simulink library "Collector_Unglazed_ISO_2node"  (R2018b)
settings: Solver=ode45  StartTime=0.0  StopTime=10.0  RelTol=1e-3  EnableMultiTasking=on
undefined symbols (not defined in the file): path_carnot
libraries: carnot x5
settings Model: Creator=drhf  LastModifiedBy=drhf
settings DataIOCC: LimitDataPoints=on  SaveFormat=Array  SignalLoggingSaveFormat=ModelDataLogs
settings OptimizationCC: ExpressionDepthLimit=2147483647  LifeSpan=inf
settings DebuggingCC: UnderspecifiedInitializationDetection=Classic  MergeDetectMultiDrivingBlocksExec=none  SolverPrmCheckMsg=warning  FcnCallInpInsideContextMsg=warning  StateNameClashWarn=warning  SFUnexpectedBacktrackingDiag=warning  SFNoUnconditionalDefaultTransitionDiag=warning  SFExecutionAtInitializationDiag=none
settings HardwareCC: ProdBitPerPointer=32  ProdBitPerSizeT=32  ProdBitPerPtrDiffT=32  ProdLargestAtomicFloat=None  ProdIntDivRoundTo=Undefined  ProdEndianess=Unspecified  ProdWordSize=32  ProdHWDeviceType=32-bit Generic
settings ModelReferenceCC: PropagateSignalLabelsOutOfModel=off
settings SFSimCC: SimUseLocalCustomCode=off
settings RTWCC: RTWUseLocalCustomCode=off
settings CodeAppCC: StateflowObjectComments=on
settings GRTTargetCC: TargetLangStandard=C89/C90 (ANSI)  GeneratePreprocessorConditionals=Disable all  CombineOutputUpdateFcns=off  GRTInterface=on
settings ConfigComp: CovMetricSettings=dw  CovHtmlReporting=on  CovSaveCumulativeToWorkspaceVar=on  CovSaveSingleToWorkspaceVar=on  CovExternalEMLEnable=off

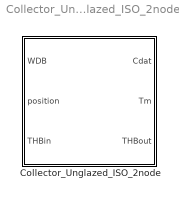
== system Collector_Unglazed_ISO_2node ==
  Collector_Unglazed_ISO_2node : Subsystem  mask(Unglazed solar thermal collector){tini=20, Ncollector=1, PathName=fullfile(path_carnot('libsl'), 'Source', 'Solar_Thermal', 'Collector_Unglazed_ISO9806', 'parameter_set'), FileName='Viessmann_SLK_ISO9806.mat', userPath=off, userParam=off, acol=2.544, len=2.1, eta0=0.702, bu=0.066, b1=32.64, b2=3.59, c_abs=50*3900, dplin=5504.4, dpqua=6222.096}
      mask prompts: tini "Initial temperature [°C]"; Ncollector "Number of collectors in parallel"; PathName "Path"; FileName "Parameter set"; userPath "Edit path and name of parameter set"; userParam "User defined parameters"; acol "Collector surface (aperture) in [m²]"; len "Length between inlet and outlet [m]"; eta0 "Optical efficiency Eta0 [-]"; bu "bu: wind dependancy of optical efficiency in W/(m²*m/s)"; b1 "b1: heat transfer for losses [W/(m²*K)]"; b2 "b2: wind dependent heat transfer for losses [W/(m²*K*m/s)]"; c_abs "Effective heat capacity of absorber [J/(m²*K)]"; dplin "Linear pressure drop in Pa/(kg/s)"; dpqua "Quadratic pressure drop in Pa/(kg/s)²"
      mask help:
      | Modified ISO 9806 model of an unglazed solar thermal collector with 2 thermal capacity nodes. The first thermal node is at the inlet, the second node is at the oulet. Both nodes have half of the capacity of the ISO test report.
      |  Qdot = A*G*(eta0*(1-bu*vwind) - (b1 + b2*vwind)*(Tm-Tamb)/G)
      |  Qdot = mdot*cp*(Tout-Tin)
      |  Tm = (Tout+Tin)/2
      |  dTin/dt = mdot*cp*(Tinlet-Tin)*2/(Acol*Ncol*CapAbs)
      |  dTout/dt = (-mdot*cp*(Tout-Tin)/(Acol*Ncol) + (G*eta0*(1-bu*vwind) - (b1 + b2*vwind)*(Tm-Tamb)))*2/CapAbs
      | This modified equations respect energy conservation also for variable inlet conditions (e.g. temperature).
      | IT IS RECOMMENDED TO USE THIS MODEL FOR SYSTEM SIMULATIONS (instead of the Collector Unglazed ISO 9806 model).
      mask init:
      | % callback to set parameters of model
      | [ok, param] = CarnotCallbacks_CONFblocksMain('SetParameters',gcbh,PathName,FileName, ...
      |     fullfile('Source','Solar_Thermal','Collector_Unglazed_ISO_2node','parameter_set'));
      | 
      | % [ok, param] = CarnotCallbacks_CollectorUnglazedConf('SetParameters',gcbh,PathName,FileName);
      mask Help: web(fullfile(path_carnot('help'),'Collector_Unglazed_ISO_2node.html'),'-helpbrowser')
      mask TypeOptions tini: Integrator/InitialCondition | Tin_node/Integrator/InitialCondition
      mask TypeOptions Ncollector: ncol/Gain | Pressure Drop/Ncoll/Value
      mask Callback userPath:
      | [ok, param] = CarnotCallbacks_CONFblocksMain('UserEdit',gcbh,...
      |     'userPath','userParam','FileName');
      mask Callback userParam: [ok, param] = CarnotCallbacks_CONFblocksMain('UserEdit',gcbh,'userPath','userParam','FileName');
      mask TypeOptions acol: acol/Value
      mask TypeOptions len: Pressure Drop/Pressure_Drop_Collector/len
      mask TypeOptions eta0: eta0/Gain
      mask TypeOptions bu: bu/Gain
      mask TypeOptions b1: b1/Bias
      mask TypeOptions b2: b2/Gain
      mask TypeOptions c_abs: c_abs/Value
      mask TypeOptions dplin: Pressure Drop/Pressure_Drop_Collector/lin
      mask TypeOptions dpqua: Pressure Drop/Pressure_Drop_Collector/qua
      mask DialogControl Container7 Prompt: Calculation
      mask DialogControl ParameterGroupVar Prompt: Picking a parameter set
      mask DialogControl Control3 Prompt: Carnot public data
      mask DialogControl Control3 Callback:
      | [ok,file] = CarnotCallbacks_CONFblocksMain('GetFilename',gcbh, 'public', ...
      |     fullfile('Source','Solar_Thermal','Collector_Unglazed_ISO_2node','parameter_set'), ...
      |     'userPath','userParam','PathName','FileName');
      mask DialogControl Control4 Prompt: Carnot internal data
      mask DialogControl Control4 Callback:
      | [ok,file] = CarnotCallbacks_CONFblocksMain('GetFilename',gcbh, 'internal', ...
      |     fullfile('Source','Solar_Thermal','Collector_Unglazed_ISO_2node','parameter_set'), ...
      |     'userPath','userParam','PathName','FileName');
      mask DialogControl Control2 Prompt: Selected path
      mask DialogControl Control2 Callback:
      | [ok,file] = CarnotCallbacks_CONFblocksMain('GetFilename',gcbh, 'selected', ...
      |     fullfile('Source','Solar_Thermal','Collector_Unglazed_ISO_2node','parameter_set'), ...
      |     'userPath','userParam','PathName','FileName');
      mask DialogControl Container9 Prompt: Parameter values
      mask DialogControl Container8 Prompt: Geometry
      mask DialogControl Container11 Prompt: Thermal
      mask DialogControl Container12 Prompt: Hydraulic
      mask DialogControl Control6 Prompt: Save in Carnot internal data
      mask DialogControl Control6 Callback:
      | [ok, param] = CarnotCallbacks_CONFblocksMain('SaveFilename',gcbh,'internal','USTC', ...
      |     fullfile('Source','Solar_Thermal','Collector_Unglazed_ISO_2node','parameter_set'), ...
      |     'userPath','userParam','PathName','FileName');
      mask DialogControl Control5 Prompt: Save in selected path
      mask DialogControl Control5 Callback:
      | [ok, param] = CarnotCallbacks_CONFblocksMain('SaveFilename',gcbh,'selected','USTC', ...
      |     fullfile('Source','Solar_Thermal','Collector_Unglazed_ISO_2node','parameter_set'), ...
      |     'userPath','userParam','PathName','FileName');
      mask Display:
      | % user defined picture file
      | picfile = fullfile(path_carnot('intlibsl'), ...
      |     'Source','Solar_Thermal','Collector_Unglazed_ISO_2node','parameter_set','Collector_CONF.jpg');
      | 
      | pic = false;
      | 
      | % show internal picture if defined
      | if ~BlockIsInCarnotLibrary    % if not located in library any more
      |     if exist(picfile)
      |         image(imread(picfile), [0.2, 0, 0.6, 1])
      |         set_param(gcb, 'BackgroundColor', 'White')
      |         pic = true;
      |     end
      | end
      | 
      | if ~pic % show public picture
      |     disp('ISO unglazed 2 node\n\n\n\n\n\n\n\n\n\n')
      |     plot([0,70,70,0,0]/140+0.1,         [-0,-0,5,5,-0]/140+0.1, ...
      |         [30,30,100,100,30]/140+0.1,     [100,94,94,100,100]/140+0.1, ...
      |         [32,1]/140+0.1,                 [94,5]/140+0.1, ...
      |         [40,10]/140+0.1,                [94,5]/140+0.1, ...
      |         [49,19]/140+0.1,                [94,5]/140+0.1, ...
      |         [57,27]/140+0.1,                [94,5]/140+0.1, ...
      |         [65,35]/140+0.1,                [94,5]/140+0.1, ...
      |         [73,43]/140+0.1,                [94,5]/140+0.1, ...
      |         [82,51]/140+0.1,                [94,5]/140+0.1, ...
      |         [90,60]/140+0.1,                [94,5]/140+0.1,...
      |         [98,68]/140+0.1,                [94,5]/140+0.1)
      |     set_param(gcb, 'BackgroundColor', 'Yellow')
      | end

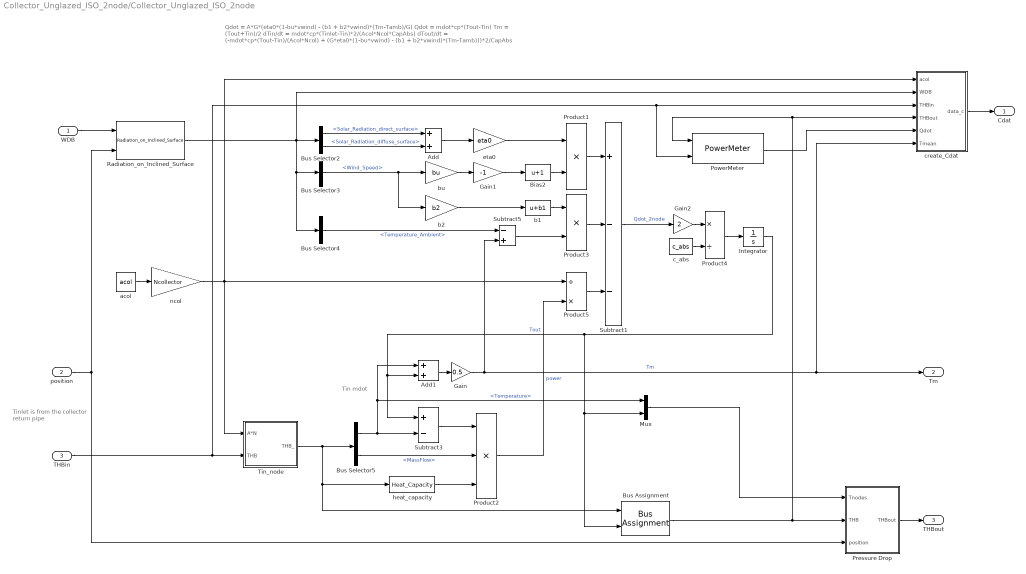
== system Collector_Unglazed_ISO_2node/Collector_Unglazed_ISO_2node ==
  note: Qdot = A*G*(eta0*(1-bu*vwind) - (b1 + b2*vwind)*(Tm-Tamb)/G)
      | Qdot = mdot*cp*(Tout-Tin)
      | Tm = (Tout+Tin)/2
      | dTin/dt = mdot*cp*(Tinlet-Tin)*2/(Acol*Ncol*CapAbs)
      | dTout/dt = (-mdot*cp*(Tout-Tin)/(Acol*Ncol) + (G*eta0*(1-bu*vwind) - (b1 + b2*vwind)*(Tm-Tamb)))*2/CapAbs
  note: Tin
      | mdot
  note: Tinlet is from the
      | collector return pipe
  WDB : Inport
  position : Inport  Port=2
  THBin : Inport  Port=3
  Add : Sum  Inputs=2
  Add1 : Sum
  Bias2 : Bias  Bias=1
  Bus Assignment : BusAssignment  AssignedSignals=Temperature
  Bus Selector2 : BusSelector  OutputSignals=Solar_Radiation_direct_surface,Solar_Radiation_diffuse_surface
  Bus Selector3 : BusSelector  OutputSignals=Wind_Speed
  Bus Selector4 : BusSelector  OutputSignals=Temperature_Ambient
  Bus Selector5 : BusSelector  OutputSignals=Temperature,MassFlow
  Gain : Gain  Gain=0.5
  Gain1 : Gain  Gain=-1
  Gain2 : Gain  Gain=2
  Integrator : Integrator  InitialCondition=tini
  Mux : Mux  Inputs=2
  PowerMeter : carnot/Control/PowerMeter
      settings: SourceProductName=Carnot
  Pressure Drop : Subsystem
  Product1 : Product  RndMeth=Zero
  Product2 : Product  Inputs=3  RndMeth=Zero
  Product3 : Product  RndMeth=Zero
  Product4 : Product  Inputs=*/  RndMeth=Zero
  Product5 : Product  Inputs=/*  RndMeth=Zero
  Radiation_on_Inclined_Surface : carnot/Weather/Radiation_on_Inclined_Surface  sky=Perez 1990  reflect=0.2
      settings: SourceProductName=Carnot
  Subtract1 : Sum  Inputs=+--
  Subtract3 : Sum  Inputs=+-
  Subtract5 : Sum  Inputs=-+
  Tin_node : Subsystem
  acol : Constant  Value=acol
  b1 : Bias  Bias=b1
  b2 : Gain  Gain=b2
  bu : Gain  Gain=bu
  c_abs : Constant  Value=c_abs
  create_Cdat : Subsystem
  eta0 : Gain  Gain=eta0
  heat_capacity : carnot/Basic/Material_Properties/Heat_Capacity  VariantControl=CarlibClassic  INPUTARGUMENTS=THB  DEBUGLEVEL=DEBUGLEVEL  MAXTOTALWARNINGS=inf  MAXCONSECUTIVEWARNINGS=inf  WRITETOFILE=0  FILENAME='errors.txt'
      settings: SourceProductName=Carnot
  ncol : Gain  Gain=Ncollector
  Cdat : Outport
  Tm : Outport  Port=2
  THBout : Outport  Port=3  InitialOutput=0
  wires:
  Gain2/1 -> Product4/1
  Mux/1 -> Pressure Drop/1(Tnodes)
  Gain/1 -> Tm/1, create_Cdat/6(Tmean), Subtract5/2  "Tm"
  Add1/1 -> Gain/1
  Integrator/1 -> Mux/2, Bus Assignment/2, Add1/2, Subtract3/1  "Tout"
  THBin/1 -> Tin_node/2(THB), PowerMeter/2, create_Cdat/3(THBin)
  Tin_node/1(THB_) -> Bus Assignment/1, heat_capacity/1, Bus Selector5/1
  Pressure Drop/1(THBout) -> THBout/1
  Product1/1 -> Subtract1/1
  Bus Selector4/1 -> Subtract5/1  "<Temperature_Ambient>"
  Bus Selector2/1 -> Add/1  "<Solar_Radiation_direct_surface>"
  Bus Selector5/1 -> Add1/1, Mux/1, Subtract3/2  "<Temperature>"
  Bus Selector2/2 -> Add/2  "<Solar_Radiation_diffuse_surface>"
  heat_capacity/1 -> Product2/3
  b2/1 -> b1/1
  Product3/1 -> Subtract1/2
  eta0/1 -> Product1/1
  Subtract5/1 -> Product3/2
  Bus Selector3/1 -> bu/1, b2/1  "<Wind_Speed>"
  b1/1 -> Product3/1
  Add/1 -> eta0/1
  Bias2/1 -> Product1/2
  Radiation_on_Inclined_Surface/1 -> Bus Selector2/1, Bus Selector3/1, Bus Selector4/1, create_Cdat/2(WDB)
  Product5/1 -> Subtract1/3
  Bus Selector5/2 -> Product2/2  "<MassFlow>"
  Subtract3/1 -> Product2/1
  Product2/1 -> Product5/2  "power"
  WDB/1 -> Radiation_on_Inclined_Surface/1
  create_Cdat/1(data_c) -> Cdat/1
  Product4/1 -> Integrator/1
  Subtract1/1 -> Gain2/1  "Qdot_2node"
  position/1 -> Pressure Drop/3(position), Radiation_on_Inclined_Surface/2
  c_abs/1 -> Product4/2
  acol/1 -> ncol/1
  bu/1 -> Gain1/1
  Bus Assignment/1 -> Pressure Drop/2(THB), create_Cdat/4(THBout), PowerMeter/1
  ncol/1 -> Tin_node/1(A*N), create_Cdat/1(acol), Product5/1
  Gain1/1 -> Bias2/1
  PowerMeter/1 -> create_Cdat/5(Qdot)

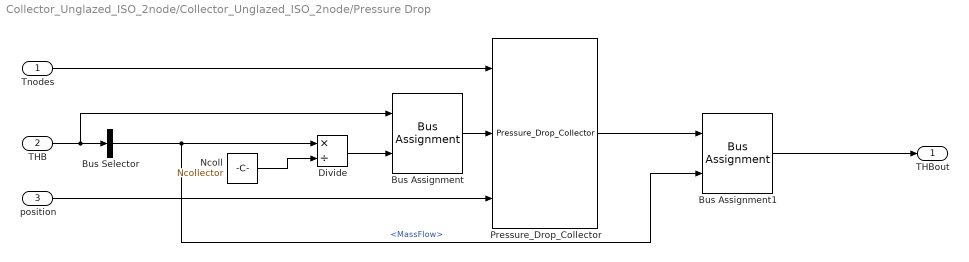
== system Collector_Unglazed_ISO_2node/Collector_Unglazed_ISO_2node/Pressure Drop ==
  Tnodes : Inport
  THB : Inport  Port=2
  position : Inport  Port=3
  Bus Assignment : BusAssignment  AssignedSignals=MassFlow
  Bus Assignment1 : BusAssignment  AssignedSignals=MassFlow
  Bus Selector : BusSelector  OutputSignals=MassFlow
  Divide : Product  Inputs=*/
  Ncoll : Constant  Value=Ncollector
  Pressure_Drop_Collector : carnot/Basic/Pressure_Drop/Pressure_Drop_Collector  len=len  lin=dplin  qua=dpqua
      settings: SourceProductName=Carnot
  THBout : Outport
  wires:
  Bus Assignment1/1 -> THBout/1
  Ncoll/1 -> Divide/2
  Divide/1 -> Bus Assignment/2
  Bus Selector/1 -> Bus Assignment1/2, Divide/1  "<MassFlow>"
  Bus Assignment/1 -> Pressure_Drop_Collector/2
  Pressure_Drop_Collector/1 -> Bus Assignment1/1
  Tnodes/1 -> Pressure_Drop_Collector/1
  position/1 -> Pressure_Drop_Collector/3
  THB/1 -> Bus Selector/1, Bus Assignment/1

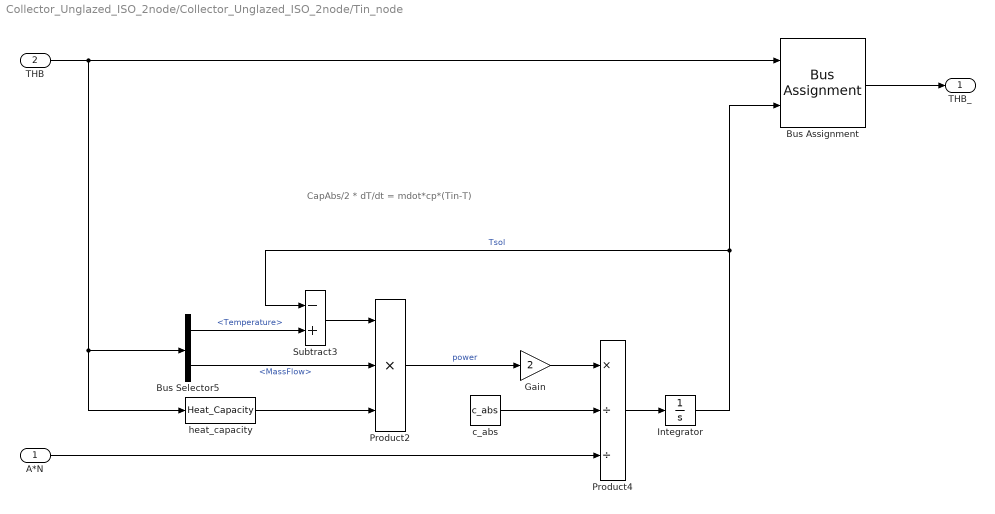
== system Collector_Unglazed_ISO_2node/Collector_Unglazed_ISO_2node/Tin_node ==
  note: CapAbs/2 * dT/dt = mdot*cp*(Tin-T)
  A*N : Inport
  THB : Inport  Port=2
  Bus Assignment : BusAssignment  AssignedSignals=Temperature
  Bus Selector5 : BusSelector  OutputSignals=Temperature,MassFlow
  Gain : Gain  Gain=2
  Integrator : Integrator  InitialCondition=tini
  Product2 : Product  Inputs=3  RndMeth=Zero
  Product4 : Product  Inputs=*//  RndMeth=Zero
  Subtract3 : Sum  Inputs=-+
  c_abs : Constant  Value=c_abs
  heat_capacity : carnot/Basic/Material_Properties/Heat_Capacity  VariantControl=CarlibClassic  INPUTARGUMENTS=THB  DEBUGLEVEL=DEBUGLEVEL  MAXTOTALWARNINGS=inf  MAXCONSECUTIVEWARNINGS=inf  WRITETOFILE=0  FILENAME='errors.txt'
      settings: SourceProductName=Carnot
  THB_ : Outport
  wires:
  A*N/1 -> Product4/3
  c_abs/1 -> Product4/2
  Integrator/1 -> Subtract3/1, Bus Assignment/2  "Tsol"
  Gain/1 -> Product4/1
  Product2/1 -> Gain/1  "power"
  Subtract3/1 -> Product2/1
  Bus Selector5/2 -> Product2/2  "<MassFlow>"
  Bus Selector5/1 -> Subtract3/2  "<Temperature>"
  heat_capacity/1 -> Product2/3
  Bus Assignment/1 -> THB_/1
  THB/1 -> Bus Assignment/1, Bus Selector5/1, heat_capacity/1
  Product4/1 -> Integrator/1

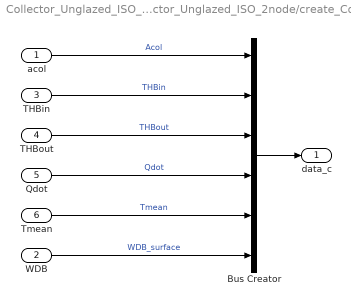
== system Collector_Unglazed_ISO_2node/Collector_Unglazed_ISO_2node/create_Cdat ==
  acol : Inport
  WDB : Inport  Port=2
  THBin : Inport  Port=3
  THBout : Inport  Port=4
  Qdot : Inport  Port=5
  Tmean : Inport  Port=6
  Bus Creator : BusCreator  Inputs=6
  data_c : Outport
  wires:
  Tmean/1 -> Bus Creator/5  "Tmean"
  Qdot/1 -> Bus Creator/4  "Qdot"
  Bus Creator/1 -> data_c/1
  WDB/1 -> Bus Creator/6  "WDB_surface"
  THBout/1 -> Bus Creator/3  "THBout"
  THBin/1 -> Bus Creator/2  "THBin"
  acol/1 -> Bus Creator/1  "Acol"
